simulink model "proj_model"  (R2025b)
settings: Solver=VariableStepDiscrete  StartTime=0.0  StopTime=10  FixedStep=0.2  RelTol=1e-3
libraries: hdlsllib x3, simulink x2
settings Model: Creator=vladc  LastModifiedBy=vladc
settings OptimizationCC: BlockReduction=off  ConditionallyExecuteInputs=off
settings DebuggingCC: SingleTaskRateTransMsg=error

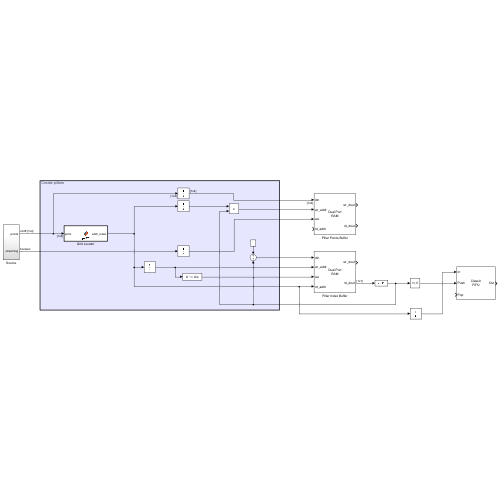
[thumbnail: Simulink's stored preview of the top-level diagram]
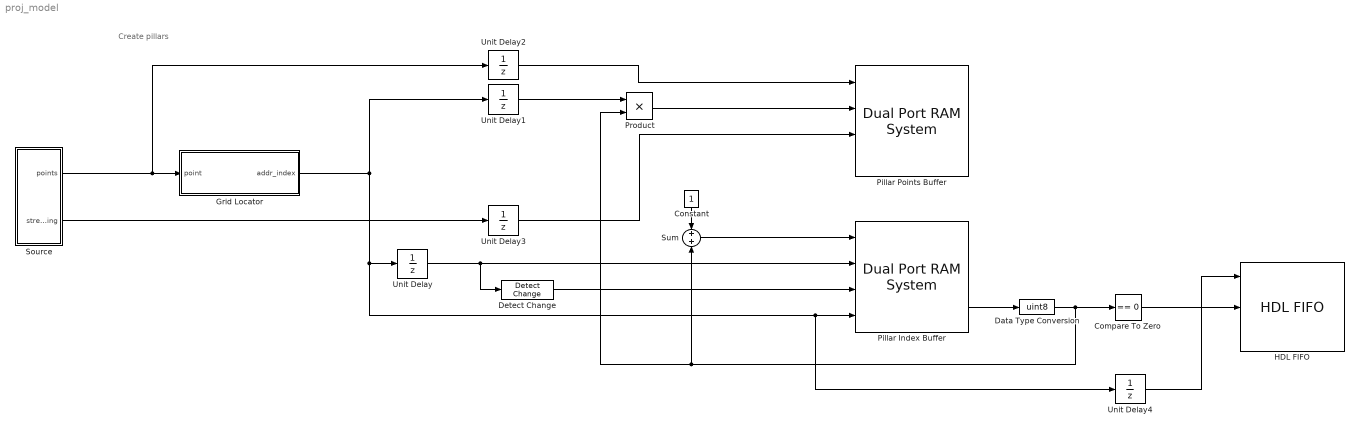
== system proj_model ==
  note: Create pillars
  Compare To Zero : simulink/Logic and Bit Operations/Compare To Zero  relop===  OutDataTypeStr=boolean
  Constant : Constant  OutDataTypeStr=uint16
  Data Type Conversion : DataTypeConversion  OutDataTypeStr=uint8  SaturateOnIntegerOverflow=off  RndMeth=Floor
  Detect Change : simulink/Logic and Bit Operations/Detect Change  vinit=0  OutDataTypeStr=boolean
      settings: LibrarySourceBlock=|
      | hdlsllib/Logic and Bit
      | Operations/Detect
      | Change
  Grid Locator : MATLAB Function  TreatAsAtomicUnit=on
  HDL FIFO : hdlsllib/HDL RAMs/HDL FIFO  fifo_size=512  mode=Classic  ratio=1  push_msg=Warning  pop_msg=Warning  show_empty=off  show_full=off  show_num=off  LabelModeActiveChoice_Mode=Classic  rst_port=off
  Pillar Index Buffer : hdlsllib/HDL RAMs/Dual Port RAM System  RAMType=Dual port  AsyncRead=off  WriteOutputValue=New data  RAMInitialValue=0  allowBusInputs=off  WritesHaveOutput=on  NumReads=0  NumWrites=1  SimulateUsing=Code generation  ModelRAMDelay=on  VectorAccess=Parallel
  Pillar Points Buffer : hdlsllib/HDL RAMs/Dual Port RAM System  RAMType=Dual port  AsyncRead=off  WriteOutputValue=New data  RAMInitialValue=0  allowBusInputs=off  WritesHaveOutput=on  NumReads=0  NumWrites=1  SimulateUsing=Code generation  ModelRAMDelay=on  VectorAccess=Parallel
  Product : Product
  Source : Subsystem
  Sum : Sum
  Unit Delay{,1..4} (5 alike) : UnitDelay  SampleTime=-1  HasFrameUpgradeWarning=on
  wires:
  Pillar Index Buffer/2 -> Data Type Conversion/1
  Sum/1 -> Pillar Index Buffer/1
  Unit Delay/1 -> Pillar Index Buffer/2, Detect Change/1
  Detect Change/1 -> Pillar Index Buffer/3
  Grid Locator/1(addr_index) -> Unit Delay4/1, Pillar Index Buffer/4, Unit Delay/1, Unit Delay1/1
  Constant/1 -> Sum/1
  Source/1(points) -> Grid Locator/1(point), Unit Delay2/1
  Data Type Conversion/1 -> Product/2, Sum/2, Compare To Zero/1
  Unit Delay1/1 -> Product/1
  Product/1 -> Pillar Points Buffer/2
  Unit Delay2/1 -> Pillar Points Buffer/1
  Source/2(streaming) -> Unit Delay3/1
  Unit Delay3/1 -> Pillar Points Buffer/3
  Compare To Zero/1 -> HDL FIFO/2
  Unit Delay4/1 -> HDL FIFO/1

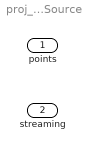
== system proj_model/Source ==
  points : Outport  OutDataTypeStr=uint8  PortDimensions=[1, 4]  SampleTime=0.2
  streaming : Outport  Port=2  OutDataTypeStr=boolean  SampleTime=0.2

== matlab function proj_model/Grid Locator ==
  data: point input; addr_index output
function addr_index = getXY(point)
%#codegen
arguments
    point (1, 4) uint8
end

x = point(1);
y = point(2);

addr_index = y * 256 + x;
